simulink model "CIC"  (R2023b)
settings: Solver=FixedStepAuto  StartTime=0.0  StopTime=1  FixedStep=1/Fs  RelTol=1e-3
undefined symbols (not defined in the file or in its folder): D, Fs, NN
settings Model: Creator=mpolj  LastModifiedBy=mpolj

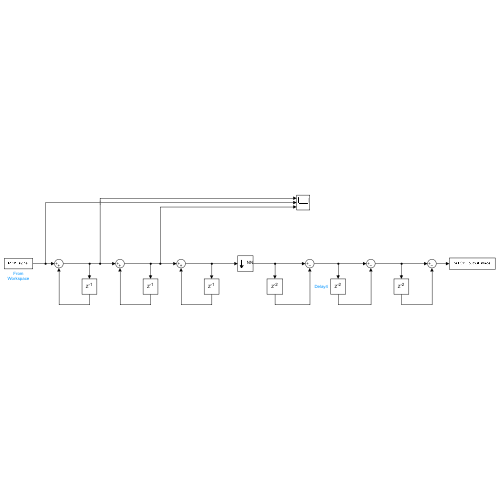
[thumbnail: Simulink's stored preview of the top-level diagram]
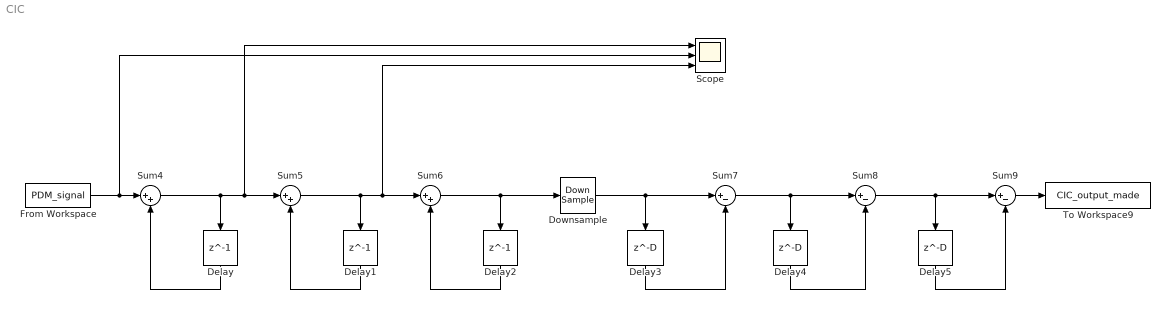
== system CIC ==
  Delay : Delay  DelayLength=1  InitialCondition=0
  Delay1 : Delay  DelayLength=1  InitialCondition=0
  Delay2 : Delay  DelayLength=1  InitialCondition=0
  Delay3 : Delay  DelayLength=D  InitialCondition=0  SampleTime=NN/Fs
  Delay4 : Delay  DelayLength=D  InitialCondition=0  SampleTime=NN/Fs
  Delay5 : Delay  DelayLength=D  InitialCondition=0  SampleTime=NN/Fs
  Downsample : DownSample  N=NN  AllowArbitraryFixedInput=on
  From Workspace : FromWorkspace  VariableName=PDM_signal
  Scope : Scope  NumInputPorts=3
  Sum4 : Sum  Inputs=|++
  Sum5 : Sum  Inputs=|++
  Sum6 : Sum  Inputs=|++
  Sum7 : Sum  Inputs=|+-
  Sum8 : Sum  Inputs=|+-
  Sum9 : Sum  Inputs=|+-
  To Workspace9 : ToWorkspace  VariableName=CIC_output_made  SaveFormat=Timeseries  SampleTime=NN/Fs
  wires:
  Sum6/1 -> Downsample/1, Delay2/1
  From Workspace/1 -> Scope/2, Sum4/1
  Delay4/1 -> Sum8/2
  Downsample/1 -> Sum7/1, Delay3/1
  Sum7/1 -> Delay4/1, Sum8/1
  Sum8/1 -> Sum9/1, Delay5/1
  Delay5/1 -> Sum9/2
  Delay3/1 -> Sum7/2
  Delay2/1 -> Sum6/2
  Sum4/1 -> Sum5/1, Scope/1, Delay/1
  Delay1/1 -> Sum5/2
  Delay/1 -> Sum4/2
  Sum5/1 -> Sum6/1, Scope/3, Delay1/1
  Sum9/1 -> To Workspace9/1
